simulink library "Pressure_Drop_Collector"  (Simulink 8.2)
settings: Solver=ode45  StartTime=0.0  StopTime=10.0  RelTol=1e-3
libraries: carnot x2, simulink_extras x1
settings Model: Creator=drhf  LastModifiedBy=drhf

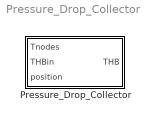
== system Pressure_Drop_Collector ==
  Pressure_Drop_Collector : Subsystem  mask(Pressure Drop Collector){len=1, lin=10, qua=10}
      mask prompts: len "Length of Collector"; lin "lin: linear pressure drop in Pa/(kg/s)"; qua "qua: quadratic pressure drop in Pa/(kg/s)²"
      mask help:
      | Calculates the pressure drop according to constant values of con, lin and qua:
      | dp_dyn = con + lin*mdot + qua*mdot²
      | Static height is taken in account via the collector inclination, the length and the temperatures:
      | dp_stat = density * grav * height
      | Total pressure is dp = dp_dyn + dpstat
      mask Help: web(fullfile(path_carnot('help'),'Pressure_Drop_Collector.html'),'-helpbrowser')

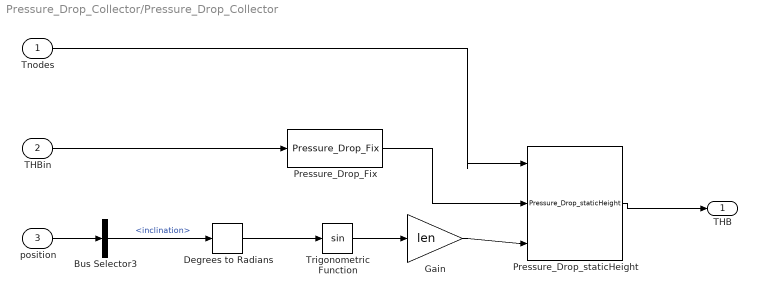
== system Pressure_Drop_Collector/Pressure_Drop_Collector ==
  Tnodes : Inport
  THBin : Inport  Port=2
  position : Inport  Port=3
  Bus Selector3 : BusSelector  OutputSignals=inclination
  Degrees to Radians : simulink_extras/Transformations/Degrees to Radians
  Gain : Gain  Gain=len
  Pressure_Drop_Fix : carnot/Basic/Pressure_Drop/Pressure_Drop_Fix  con=0  lin=lin  qua=qua
  Pressure_Drop_staticHeight : carnot/Basic/Pressure_Drop/Pressure_Drop_staticHeight
  Trigonometric Function : Trigonometry
  THB : Outport
  wires:
  Bus Selector3/1 -> Degrees to Radians/1  "<inclination>"
  position/1 -> Bus Selector3/1
  Trigonometric Function/1 -> Gain/1
  THBin/1 -> Pressure_Drop_Fix/1
  Pressure_Drop_Fix/1 -> Pressure_Drop_staticHeight/2
  Tnodes/1 -> Pressure_Drop_staticHeight/1
  Pressure_Drop_staticHeight/1 -> THB/1
  Gain/1 -> Pressure_Drop_staticHeight/3
  Degrees to Radians/1 -> Trigonometric Function/1
